simulink model "Inverted_pendulum_Simulink_with_PIDcontrol"  (R2017a)
settings: Solver=VariableStepAuto  StartTime=0.0  StopTime=10  RelTol=1e-3
values from neighbouring files (symbols this model uses):
  b = 0.1    [Inverted_Pendulum_State_Space.m]    (also in Inverted_Pendulum_Transfer_Function.m)
  g = 9.8    [Inverted_Pendulum_State_Space.m]    (also in Inverted_Pendulum_Transfer_Function.m)
  I = 0.006    [Inverted_Pendulum_State_Space.m]    (also in Inverted_Pendulum_Transfer_Function.m)
  L = 0.3    [Inverted_Pendulum_State_Space.m]    (also in Inverted_Pendulum_Transfer_Function.m)
  m = 0.2    [Inverted_Pendulum_State_Space.m]    (also in Inverted_Pendulum_Transfer_Function.m)
  M = 0.5    [Inverted_Pendulum_State_Space.m]    (also in Inverted_Pendulum_Transfer_Function.m)
libraries: simulink x1
settings Model: Creator=Majed  LastModifiedBy=Majed
settings SolverCC: AlgebraicLoopSolver=LineSearch
settings DebuggingCC: AlgebraicLoopMsg=none

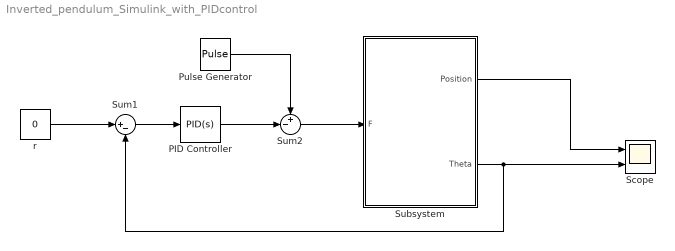
== system Inverted_pendulum_Simulink_with_PIDcontrol ==
  PID Controller : simulink/Continuous/PID Controller  Controller=PID  TimeDomain=Continuous-time  SampleTime=-1  IntegratorMethod=Forward Euler  FilterMethod=Forward Euler  Form=Parallel  UseFilter=on  ControllerParametersSource=internal  P=100  I=1  D=20  N=100  InitialConditionSource=internal  InitialConditionForIntegrator=0  InitialConditionForFilter=0  ExternalReset=none  LimitOutput=off  UpperSaturationLimit=inf  LowerSaturationLimit=-inf  LinearizeAsGain=on  AntiWindupMode=none  Kb=1  TrackingMode=off  Kt=1  PParamMin=[]  PParamMax=[]  IParamMin=[]  IParamMax=[]  DParamMin=[]  DParamMax=[]  NParamMin=[]  NParamMax=[]  KbParamMin=[]  KbParamMax=[]  KtParamMin=[]  KtParamMax=[]  POutMin=[]  POutMax=[]  IOutMin=[]  IOutMax=[]  DOutMin=[]  DOutMax=[]  NOutMin=[]  NOutMax=[]  KbOutMin=[]  KbOutMax=[]  KtOutMin=[]  KtOutMax=[]  IntegratorOutMin=[]  IntegratorOutMax=[]  FilterOutMin=[]  FilterOutMax=[]  SumOutMin=[]  SumOutMax=[]  SumI1OutMin=[]  SumI1OutMax=[]  SumI2OutMin=[]  SumI2OutMax=[]  SumI3OutMin=[]  SumI3OutMax=[]  SumDOutMin=[]  SumDOutMax=[]  SaturationOutMin=[]  SaturationOutMax=[]  IntegratorContinuousStateAttributes=''  IntegratorStateMustResolveToSignalObject=off  IntegratorRTWStateStorageClass=Auto  FilterContinuousStateAttributes=''  FilterStateMustResolveToSignalObject=off  FilterRTWStateStorageClass=Auto  DifferentiatorICPrevScaledInput=0  DifferentiatorOutMin=[]  DifferentiatorOutMax=[]  InitialConditionSetting=State (most efficient)
  Pulse Generator : DiscretePulseGenerator  PulseType=Time based  Amplitude=1000  Period=10  PulseWidth=0.01
  Scope : Scope  NumInputPorts=2
  Subsystem : Subsystem
  Sum1 : Sum  Inputs=|+-
  Sum2 : Sum  Inputs=+-|
  r : Constant  Value=0  SampleTime=10
  wires:
  Subsystem/1(Position) -> Scope/1
  Subsystem/2(Theta) -> Sum1/2, Scope/2
  Pulse Generator/1 -> Sum2/1
  r/1 -> Sum1/1
  Sum1/1 -> PID Controller/1
  PID Controller/1 -> Sum2/2
  Sum2/1 -> Subsystem/1(F)

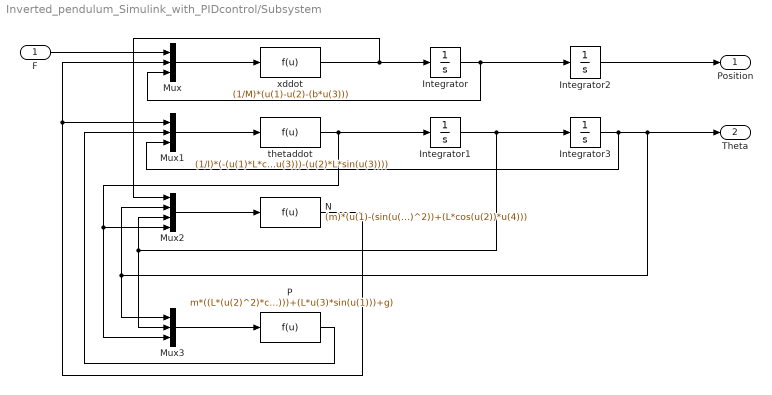
== system Inverted_pendulum_Simulink_with_PIDcontrol/Subsystem ==
  F : Inport
  Integrator : Integrator  ContinuousStateAttributes='xdot'
  Integrator1 : Integrator  ContinuousStateAttributes='Thetadot'
  Integrator2 : Integrator  ContinuousStateAttributes='x'
  Integrator3 : Integrator  InitialCondition=pi  ContinuousStateAttributes='Theta'
  Mux : Mux  Inputs=3
  Mux1 : Mux  Inputs=3
  Mux2 : Mux
  Mux3 : Mux  Inputs=3
  N : Fcn  Expr=(m)*(u(1)-(sin(u(2))*L*(u(3)^2))+(L*cos(u(2))*u(4)))
  P : Fcn  Expr=m*((L*(u(2)^2)*cos(u(1)))+(L*u(3)*sin(u(1)))+g)
  thetaddot : Fcn  Expr=(1/I)*(-(u(1)*L*cos(u(3)))-(u(2)*L*sin(u(3))))
  xddot : Fcn  Expr=(1/M)*(u(1)-u(2)-(b*u(3)))
  Position : Outport
  Theta : Outport  Port=2  Unit=rad
  wires:
  Mux1/1 -> thetaddot/1
  Mux/1 -> xddot/1
  thetaddot/1 -> Mux2/4, Mux3/3, Integrator1/1
  Mux3/1 -> P/1
  Mux2/1 -> N/1
  xddot/1 -> Mux2/1, Integrator/1
  Integrator/1 -> Mux/3, Integrator2/1
  N/1 -> Mux/2, Mux1/1
  F/1 -> Mux/1
  Integrator2/1 -> Position/1
  Integrator1/1 -> Mux2/3, Mux3/2, Integrator3/1
  P/1 -> Mux1/2
  Integrator3/1 -> Mux1/3, Theta/1, Mux3/1, Mux2/2
